simulink model "Conv2D_sim"  (R2019a)
settings: Solver=VariableStepAuto  StartTime=0.0  StopTime=10.0  RelTol=1e-3
undefined symbols (not defined in the file): conv2d_1_bias, conv2d_1_kernel, conv2d_2_bias, conv2d_2_kernel, dense_1_bias, dense_1_kernel, dense_2_bias, dense_2_kernel, X_test
settings Model: Creator=Shravan-PC  LastModifiedBy=Shravan-PC

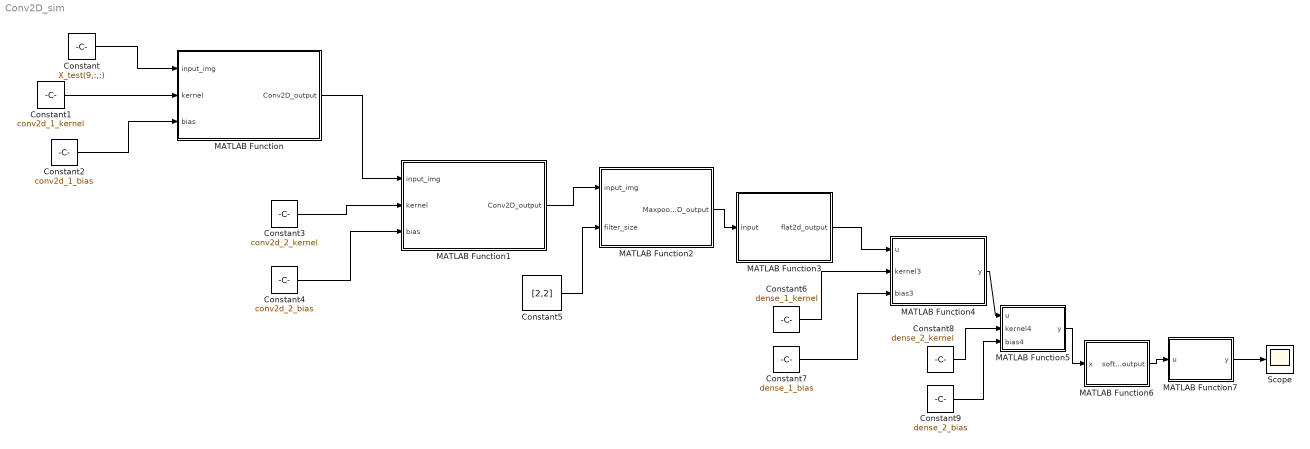
== system Conv2D_sim ==
  Constant : Constant  Value=X_test(9,:,:)
  Constant1 : Constant  Value=conv2d_1_kernel
  Constant2 : Constant  Value=conv2d_1_bias
  Constant3 : Constant  Value=conv2d_2_kernel
  Constant4 : Constant  Value=conv2d_2_bias
  Constant5 : Constant  Value=[2,2]
  Constant6 : Constant  Value=dense_1_kernel
  Constant7 : Constant  Value=dense_1_bias
  Constant8 : Constant  Value=dense_2_kernel
  Constant9 : Constant  Value=dense_2_bias
  MATLAB Function : MATLAB Function  TreatAsAtomicUnit=on  RTWFcnName=CONV2D
      settings: RTWFileNameOpts=Use function name
  MATLAB Function1 : MATLAB Function  TreatAsAtomicUnit=on  RTWFcnName=CONV2D
      settings: RTWFileNameOpts=Use function name
  MATLAB Function2 : MATLAB Function  TreatAsAtomicUnit=on
  MATLAB Function3 : MATLAB Function  TreatAsAtomicUnit=on
  MATLAB Function4 : MATLAB Function  TreatAsAtomicUnit=on
  MATLAB Function5 : MATLAB Function  TreatAsAtomicUnit=on
  MATLAB Function6 : MATLAB Function  TreatAsAtomicUnit=on
  MATLAB Function7 : MATLAB Function  TreatAsAtomicUnit=on
  Scope : Scope
  wires:
  Constant/1 -> MATLAB Function/1(input_img)
  Constant1/1 -> MATLAB Function/2(kernel)
  Constant2/1 -> MATLAB Function/3(bias)
  Constant3/1 -> MATLAB Function1/2(kernel)
  Constant4/1 -> MATLAB Function1/3(bias)
  MATLAB Function1/1(Conv2D_output) -> MATLAB Function2/1(input_img)
  Constant5/1 -> MATLAB Function2/2(filter_size)
  MATLAB Function2/1(Maxpool2D_output) -> MATLAB Function3/1(input)
  Constant6/1 -> MATLAB Function4/2(kernel3)
  Constant7/1 -> MATLAB Function4/3(bias3)
  MATLAB Function4/1(y) -> MATLAB Function5/1(u)
  Constant8/1 -> MATLAB Function5/2(kernel4)
  Constant9/1 -> MATLAB Function5/3(bias4)
  MATLAB Function5/1(y) -> MATLAB Function6/1(x)
  MATLAB Function6/1(softmax_output) -> MATLAB Function7/1(u)
  MATLAB Function7/1(y) -> Scope/1
  MATLAB Function/1(Conv2D_output) -> MATLAB Function1/1(input_img)
  MATLAB Function3/1(flat2d_output) -> MATLAB Function4/1(u)

== matlab function Conv2D_sim/MATLAB Function1 ==
  data: input_img input size=[1,26,26,32]; Conv2D_output output size=[1,24,24,64]; kernel input size=[64,32,3,3]; bias input size=[64,1]
function Conv2D_output = Conv2D_sim2(input_img,kernel,bias)
%img_size=size(input_img);
%size_of_img_size=size(img_size);
%kernel_size=size(kernel);
%bias_size=size(bias);
img_size=[1,26,26,32];
size_of_img_size=[1,4];
kernel_size=[64,32,3,3];
bias_size=[64,1];
output_size=[img_size(1), (img_size(2)-kernel_size(3)+1), (img_size(3)-kernel_size(4)+1), bias_size(1)];
Conv2D_output=zeros(output_size(1),output_size(2),output_size(3),output_size(4));

for img_no=1:output_size(1)
    for channel_no=1:output_size(4)
        for i=round(kernel_size(3)/2):output_size(2)+round(kernel_size(3)/2)-1
            for j=round(kernel_size(4)/2):output_size(3)+round(kernel_size(4)/2)-1
                if size_of_img_size(2)==4
                    temp_sum=single(zeros(kernel_size(3),kernel_size(4)));
                    for ip_channel=1:img_size(4)
                        temp_kernel=reshape(kernel(channel_no,ip_channel,:,:),[kernel_size(3),kernel_size(4)]);
                        
%                         if(i<round(kernel_size(3)/2))
%                             temp_kernel(1:i,:)=0;
%                         end
%                         if(j<round(kernel_size(4)/2))
%                             temp_kernel(:,1:j)=0;
%                         end
%                         if (i>output_size(2))
%                             temp_kernel(i-output_size(2)+round(kernel_size(3)/2):kernel_size(3),:)=0;
%                         end
%                         if (j>output_size(3))
%                             temp_kernel(:,j-output_size(3)+round(kernel_size(4)/2):kernel_size(4))=0;
%                         end
                        
                        temp_sum=temp_sum+reshape(input_img(img_no,i-round(kernel_size(3)/2)+1:i+round(kernel_size(3)/2)-1,j-round(kernel_size(4)/2)+1:j+round(kernel_size(4)/2)-1,ip_channel),[kernel_size(3),kernel_size(4)]).*temp_kernel.';
                    end
                    Conv2D_output(img_no,i-round(kernel_size(3)/2)+1,j-round(kernel_size(4)/2)+1,channel_no)=sum(sum(sum(temp_sum)))+bias(channel_no);
                else
                    temp_kernel=reshape(kernel(channel_no,1,:,:),[kernel_size(3),kernel_size(4)]);
%                     if(i<round(kernel_size(3)/2))
%                         temp_kernel(1:i,:)=0;
%                     end
%                     if(j<round(kernel_size(4)/2))
%                         temp_kernel(:,1:j)=0;
%                     end
%                     if (i>output_size(2))
%                         temp_kernel(i-output_size(2)+round(kernel_size(3)/2):kernel_size(3),:)=0;
%                     end
%                     if (j>output_size(3))
%                         temp_kernel(:,j-output_size(3)+round(kernel_size(4)/2):kernel_size(4))=0;
%                     end
                    Conv2D_output(img_no,i-round(kernel_size(3)/2)+1,j-round(kernel_size(4)/2)+1,channel_no)=bias(channel_no)+sum(sum(sum(reshape(input_img(img_no,i-round(kernel_size(3)/2)+1:i+round(kernel_size(3)/2)-1,j-round(kernel_size(4)/2)+1:j+round(kernel_size(4)/2)-1),[kernel_size(3),kernel_size(4)]).*temp_kernel.')));
                end
            end
        end
    end
end
Conv2D_output(Conv2D_output<0)=0;
end

== matlab function Conv2D_sim/MATLAB Function ==
  data: input_img input size=[1,28,28]; Conv2D_output output size=[1,26,26,32]; kernel input size=[32,1,3,3]; bias input size=[32,1]
function Conv2D_output = Conv2D_sim(input_img,kernel,bias)
%img_size=size(input_img);
%size_of_img_size=size(img_size);
%kernel_size=size(kernel);
%bias_size=size(bias);
img_size=[1,28,28];
size_of_img_size=[1,3];
kernel_size=[32,1,3,3];
bias_size=[32,1];
output_size=[img_size(1), (img_size(2)-kernel_size(3)+1), (img_size(3)-kernel_size(4)+1), bias_size(1)];
Conv2D_output=zeros(output_size(1),output_size(2),output_size(3),output_size(4));

for img_no=1:output_size(1)
    for channel_no=1:output_size(4)
        for i=round(kernel_size(3)/2):output_size(2)+round(kernel_size(3)/2)-1
            for j=round(kernel_size(4)/2):output_size(3)+round(kernel_size(4)/2)-1
                if size_of_img_size(2)==4
                    temp_sum=zeros(kernel_size(3),kernel_size(4));
                    for ip_channel=1:img_size(4)
                        temp_kernel=reshape(kernel(channel_no,ip_channel,:,:),[kernel_size(3),kernel_size(4)]);
                        
%                         if(i<round(kernel_size(3)/2))
%                             temp_kernel(1:i,:)=0;
%                         end
%                         if(j<round(kernel_size(4)/2))
%                             temp_kernel(:,1:j)=0;
%                         end
%                         if (i>output_size(2))
%                             temp_kernel(i-output_size(2)+round(kernel_size(3)/2):kernel_size(3),:)=0;
%                         end
%                         if (j>output_size(3))
%                             temp_kernel(:,j-output_size(3)+round(kernel_size(4)/2):kernel_size(4))=0;
%                         end
                        
                        temp_sum=temp_sum+reshape(input_img(img_no,i-round(kernel_size(3)/2)+1:i+round(kernel_size(3)/2)-1,j-round(kernel_size(4)/2)+1:j+round(kernel_size(4)/2)-1,ip_channel),[kernel_size(3),kernel_size(4)]).*temp_kernel.';
                    end
                    Conv2D_output(img_no,i-round(kernel_size(3)/2)+1,j-round(kernel_size(4)/2)+1,channel_no)=sum(sum(sum(temp_sum)))+bias(channel_no);
                else
                    temp_kernel=reshape(kernel(channel_no,1,:,:),[kernel_size(3),kernel_size(4)]);
%                     if(i<round(kernel_size(3)/2))
%                         temp_kernel(1:i,:)=0;
%                     end
%                     if(j<round(kernel_size(4)/2))
%                         temp_kernel(:,1:j)=0;
%                     end
%                     if (i>output_size(2))
%                         temp_kernel(i-output_size(2)+round(kernel_size(3)/2):kernel_size(3),:)=0;
%                     end
%                     if (j>output_size(3))
%                         temp_kernel(:,j-output_size(3)+round(kernel_size(4)/2):kernel_size(4))=0;
%                     end
                    Conv2D_output(img_no,i-round(kernel_size(3)/2)+1,j-round(kernel_size(4)/2)+1,channel_no)=bias(channel_no)+sum(sum(sum(reshape(input_img(img_no,i-round(kernel_size(3)/2)+1:i+round(kernel_size(3)/2)-1,j-round(kernel_size(4)/2)+1:j+round(kernel_size(4)/2)-1),[kernel_size(3),kernel_size(4)]).*temp_kernel.')));
                end
            end
        end
    end
end
Conv2D_output(Conv2D_output<0)=0;
end

== matlab function Conv2D_sim/MATLAB Function2 ==
  data: input_img input size=[1,24,24,64]; Maxpool2D_output output size=[1,12,12,64]; filter_size input size=2
function Maxpool2D_output = MaxPool2D(input_img,filter_size)
%img_size=size(input_img);
%output_size=[img_size(1), round(img_size(2)/filter_size(1)),round(img_size(3)/filter_size(2)),img_size(4)];
img_size=[1,24,24,64];
output_size=[1,12,12,64];
Maxpool2D_output=zeros(output_size(1),output_size(2),output_size(3),output_size(4));

for img_no=1:output_size(1)
    for channel_no=1:output_size(4)
        for i=1:output_size(2)
            for j=1:output_size(3)
                Maxpool2D_output(img_no,i,j,channel_no)=max(max(input_img(img_no, filter_size(1)*i-filter_size(1)+1:filter_size(1)*i, filter_size(2)*j-filter_size(2)+1:filter_size(2)*j,channel_no)));
            end
        end
    end
end
end

== matlab function Conv2D_sim/MATLAB Function3 ==
  data: input input size=[1,12,12,64]; flat2d_output output size=[1,9216]
function flat2d_output=Flatten(input)
%input_size=size(input);
%output_size=input_size(2)*input_size(3)*input_size(4);
input_size=[1,12,12,64];
output_size=9216;
flat2d_output=zeros(input_size(1),output_size);

for input_no=1:input_size(1)
    k=0;
    for i=1:input_size(2)
        for j=1:input_size(3)
            flat2d_output(input_no,k*input_size(4)+1:(k+1)*input_size(4))=reshape(input(input_no,i,j,:),[1,input_size(4)]);
            k=k+1;
        end
    end
end
end

== matlab function Conv2D_sim/MATLAB Function4 ==
  data: u input size=[1,9216]; y output size=[1,128]; kernel3 input size=[128,9216]; bias3 input size=[128,1]
function y = dense1(u,kernel3,bias3)
%inp_size=size(u);
%bias_size=size(bias3);
inp_size=[1,9216];
bias_size=[128,1];
y=zeros(inp_size(1),bias_size(1));

y(1,:)=u(1,:)*kernel3.'+bias3.';
y(y<0)=0;
end

== matlab function Conv2D_sim/MATLAB Function5 ==
  data: u input size=[1,128]; y output size=[1,10]; kernel4 input size=[10,128]; bias4 input size=[10,1]
function y = dense2(u,kernel4,bias4)
%inp_size=size(u);
%bias_size=size(bias4);
inp_size=[1,128];
bias_size=[10,1];
y=zeros(inp_size(1),bias_size(1));

y(1,:)=u(1,:)*kernel4.'+bias4.';
y(y<0)=0;
end

== matlab function Conv2D_sim/MATLAB Function6 ==
  data: x input size=[1,10]; softmax_output output size=[1,10]
function softmax_output=Softmax(x)
%input_size=size(x);
input_size=[1,10];
softmax_output=zeros(input_size);


for inp_no=1:input_size(1)
    exp_sum=0;
    for i=1:input_size(2)
        softmax_output(inp_no,i)=exp(x(inp_no,i));
        exp_sum=exp_sum+softmax_output(inp_no,i);
    end
    softmax_output(inp_no,:)=softmax_output(inp_no,:)/exp_sum;
    
end
end

== matlab function Conv2D_sim/MATLAB Function7 ==
  data: u input size=[1,10]; y output size=[1,1]
function y = fcn(u)
y=zeros(1,1);

[argvalue,y]=max(u.');
y=y-1;
end
